simulink model "model_2"  (R2022a)
settings: Solver=VariableStepAuto  StartTime=0.0  StopTime=5  RelTol=1e-3
values from neighbouring files (symbols this model uses):
  A = [-1, 0, 0, 0 ... (first row only)    [task_1.m]    (also in task_2.m; task_3.m = [0, 3, 0, 0; -3, 0,  0, 0; 0, 0, 0, 1; 0, 0, -1, 0]; task_4.m = [3, -11, -7, 5; -11, 3, -5, 7; -7, -5, 3, 11; 5, 7, 11, 3]; task_4ora.m = [5, -9, -7, 1; -9, 5,  -1, 7; -7, -1, 5, 9; 1, 7, 9, 5])
  C = [1, 0, 0, 0; 0, 1, 0, 0; 0, 0, 1, 0; 0, 0, 0, 1]    [task_1.m]    (also in task_2.m; task_3.m = [2, 0, 0, 3]; task_4.m = [2, -2, 2, 2; 2, 4, -2, 4]; task_4ora.m = [2, -2, 2, 2; -2, 4, 2, 4])
  L_1 = inv(Q)*Y    [task_3.m]
  L_2 = inv(Q)*Y    [task_3.m]
  L_3 = inv(Q)*Y    [task_3.m]
  x0 = [-7; -5; 2; 10]    [task_1.m]    (also in task_2.m; task_3.m = [5; -10; 2; -6]; task_4.m = [10; -15; 1; -5]; task_4ora.m = [10; -15; 1; -5])
  x_0 = [2; 5; -2; 10]    [task_3.m]    (also in task_4.m = [-10; 0; 0; 5]; task_4ora.m = [-10; 0; 0; 5])
settings Model: Creator=vital  LastModifiedBy=Family
settings DebuggingCC: UnconnectedInputMsg=warning  UnconnectedOutputMsg=warning  UnconnectedLineMsg=warning
settings RTWCC: DLArmComputeVersion=19.05

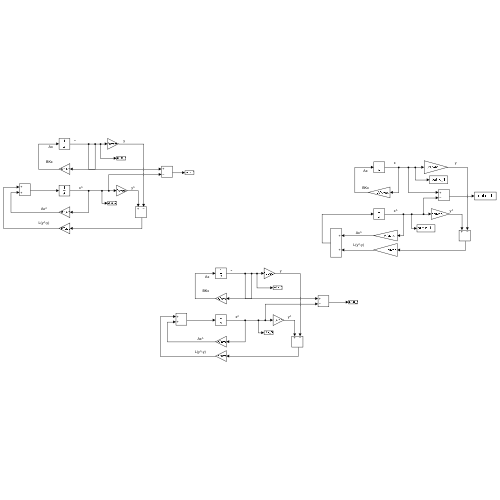
[thumbnail: Simulink's stored preview of the top-level diagram]
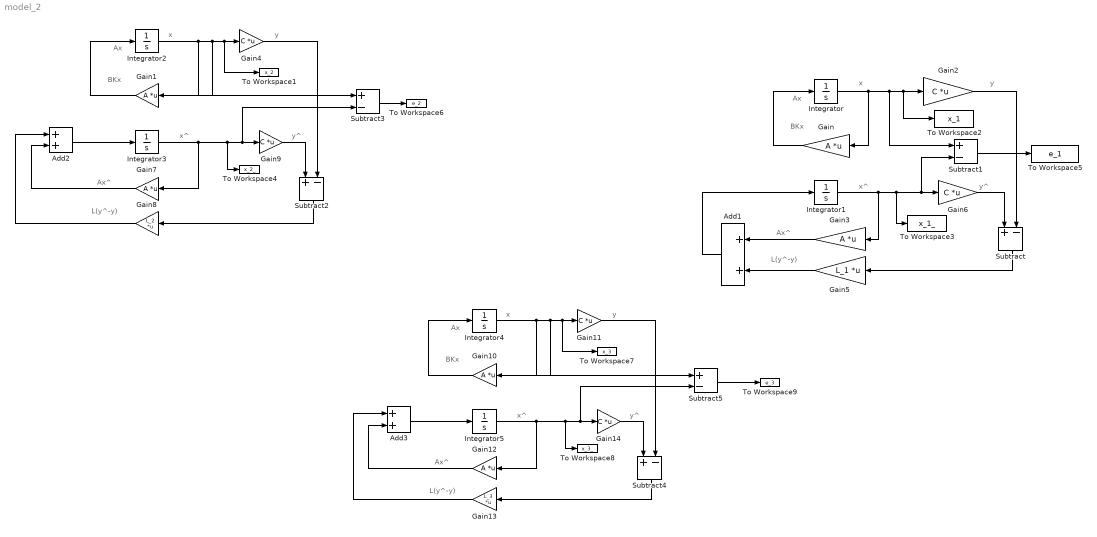
== system model_2 ==
  note: L(y^-y)
  note: Ax^
  note: y^
  note: x^
  note: y
  note: x
  note: BKx
  note: Ax
  note: y^
  note: Ax^
  note: y
  note: x^
  note: L(y^-y)
  note: BKx
  note: Ax
  note: x
  note: Ax
  note: x
  note: y
  note: y^
  note: Ax^
  note: BKx
  note: x^
  note: L(y^-y)
  Add1 : Sum
  Add2 : Sum
  Add3 : Sum
  Gain{,1,3,7,10,12} (6 alike) : Gain  Gain=A  Multiplication=Matrix(K*u) (u vector)
  Gain{2,4,6,9,11,14} (6 alike) : Gain  Gain=C  Multiplication=Matrix(K*u) (u vector)
  Gain13 : Gain  Gain=L_3  Multiplication=Matrix(K*u) (u vector)
  Gain5 : Gain  Gain=L_1  Multiplication=Matrix(K*u) (u vector)
  Gain8 : Gain  Gain=L_2  Multiplication=Matrix(K*u) (u vector)
  Integrator : Integrator  InitialCondition=x0
  Integrator1 : Integrator  InitialCondition=x_0
  Integrator2 : Integrator  InitialCondition=x0
  Integrator3 : Integrator  InitialCondition=x_0
  Integrator4 : Integrator  InitialCondition=x0
  Integrator5 : Integrator  InitialCondition=x_0
  Subtract{,1..5} (6 alike) : Sum  Inputs=+-
  To Workspace1 : ToWorkspace  VariableName=x_2  SaveFormat=Timeseries  SampleTime=0.0001
  To Workspace2 : ToWorkspace  VariableName=x_1  SaveFormat=Timeseries  SampleTime=0.0001
  To Workspace3 : ToWorkspace  VariableName=x_1_  SaveFormat=Timeseries  SampleTime=-1
  To Workspace4 : ToWorkspace  VariableName=x_2_  SaveFormat=Timeseries  SampleTime=-1
  To Workspace5 : ToWorkspace  VariableName=e_1  SaveFormat=Timeseries  SampleTime=-1
  To Workspace6 : ToWorkspace  VariableName=e_2  SaveFormat=Timeseries  SampleTime=-1
  To Workspace7 : ToWorkspace  VariableName=x_3  SaveFormat=Timeseries  SampleTime=0.0001
  To Workspace8 : ToWorkspace  VariableName=x_3_  SaveFormat=Timeseries  SampleTime=-1
  To Workspace9 : ToWorkspace  VariableName=e_3  SaveFormat=Timeseries  SampleTime=-1
  wires:
  Integrator/1 -> To Workspace2/1, Gain2/1, Subtract1/1, Gain/1
  Gain/1 -> Integrator/1
  Gain2/1 -> Subtract/2
  Add1/1 -> Integrator1/1
  Integrator1/1 -> Gain3/1, To Workspace3/1, Subtract1/2, Gain6/1
  Gain6/1 -> Subtract/1
  Subtract/1 -> Gain5/1
  Gain5/1 -> Add1/2
  Subtract1/1 -> To Workspace5/1
  Gain3/1 -> Add1/1
  Gain1/1 -> Integrator2/1
  Integrator2/1 -> To Workspace1/1, Gain4/1, Gain1/1, Subtract3/1
  Add2/1 -> Integrator3/1
  Integrator3/1 -> Gain7/1, To Workspace4/1, Subtract3/2, Gain9/1
  Gain8/1 -> Add2/1
  Subtract2/1 -> Gain8/1
  Gain4/1 -> Subtract2/2
  Gain9/1 -> Subtract2/1
  Subtract3/1 -> To Workspace6/1
  Gain7/1 -> Add2/2
  Gain12/1 -> Add3/2
  Subtract5/1 -> To Workspace9/1
  Gain11/1 -> Subtract4/2
  Subtract4/1 -> Gain13/1
  Integrator5/1 -> Gain12/1, To Workspace8/1, Subtract5/2, Gain14/1
  Gain14/1 -> Subtract4/1
  Add3/1 -> Integrator5/1
  Gain13/1 -> Add3/1
  Gain10/1 -> Integrator4/1
  Integrator4/1 -> To Workspace7/1, Gain11/1, Gain10/1, Subtract5/1
